simulink model "elevator"  (R2015b)
settings: Solver=FixedStepAuto  StartTime=0.0  StopTime=200  FixedStep=1  MaxStep=1  RelTol=1e-3
libraries: simulink x12
settings Model: Creator=DNikolaev  LastModifiedBy=DNikolaev

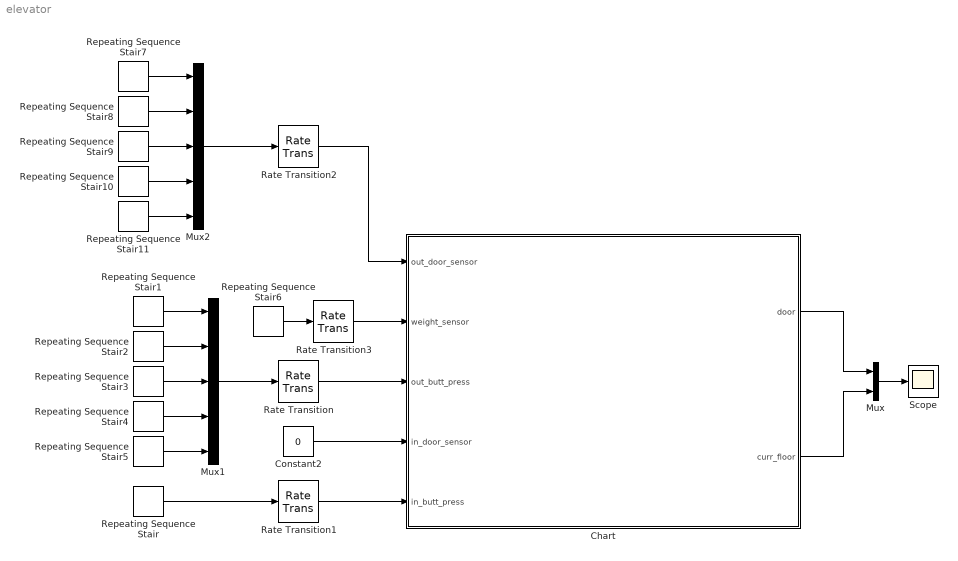
== system elevator ==
  Chart : Stateflow chart  TreatAsAtomicUnit=on
  Constant2 : Constant  Value=0
  Mux : Mux  Inputs=2
  Mux1 : Mux  Inputs=5
  Mux2 : Mux  Inputs=5
  Rate Transition{,1..3} (4 alike) : RateTransition  OutPortSampleTime=1
  Repeating Sequence Stair : simulink/Sources/Repeating Sequence Stair  OutValues=[0 0 0 4 0 0 0 0 0 1 0 0 0 0 0 0 0 0 0 0 0 0 0].'  tsamp=10  OutMin=[]  OutMax=[]  OutDataTypeStr=double  OutputDataTypeScalingMode=double  OutDataType=fixdt(0,8)  ConRadixGroup=Best Precision: Vector-wise  OutScaling=2^-12
  Repeating Sequence Stair1 : simulink/Sources/Repeating Sequence Stair  OutValues=[0 0 0 0 0 0 0 0 0 0 0 0 0 0 1 0 0 0 0 0].'  tsamp=10  OutMin=[]  OutMax=[]  OutDataTypeStr=double  OutputDataTypeScalingMode=double  OutDataType=fixdt(0,8)  ConRadixGroup=Best Precision: Vector-wise  OutScaling=2^-12
  Repeating Sequence Stair{3,5,7,9..11} (6 alike) : simulink/Sources/Repeating Sequence Stair  OutValues=[0 0 0 0 0 0 0 0 0 0 0 0 0 0 0 0 0 0 0 0].'  tsamp=10  OutMin=[]  OutMax=[]  OutDataTypeStr=double  OutputDataTypeScalingMode=double  OutDataType=fixdt(0,8)  ConRadixGroup=Best Precision: Vector-wise  OutScaling=2^-12
  Repeating Sequence Stair2 : simulink/Sources/Repeating Sequence Stair  OutValues=[0 1 0 0 0 0 0 0 0 0 0 0 0 0 0 0 0 0 0 0].'  tsamp=10  OutMin=[]  OutMax=[]  OutDataTypeStr=double  OutputDataTypeScalingMode=double  OutDataType=fixdt(0,8)  ConRadixGroup=Best Precision: Vector-wise  OutScaling=2^-12
  Repeating Sequence Stair4 : simulink/Sources/Repeating Sequence Stair  OutValues=[0 0 0 0 0 0 0 1 0 0 0 0 0 0 0 0 0 0 0 0].'  tsamp=10  OutMin=[]  OutMax=[]  OutDataTypeStr=double  OutputDataTypeScalingMode=double  OutDataType=fixdt(0,8)  ConRadixGroup=Best Precision: Vector-wise  OutScaling=2^-12
  Repeating Sequence Stair6 : simulink/Sources/Repeating Sequence Stair  OutValues=[0 0 0 50 0 0 0 0 400 400 400 200 200 0 0 0 0 0 0 0].'  tsamp=10  OutMin=[]  OutMax=[]  OutDataTypeStr=double  OutputDataTypeScalingMode=double  OutDataType=fixdt(0,8)  ConRadixGroup=Best Precision: Vector-wise  OutScaling=2^-12
  Repeating Sequence Stair8 : simulink/Sources/Repeating Sequence Stair  OutValues=[0 1 1 0 0 0 0 0 0 0 0 0 0 0 0 0 0 0 0 0].'  tsamp=10  OutMin=[]  OutMax=[]  OutDataTypeStr=double  OutputDataTypeScalingMode=double  OutDataType=fixdt(0,8)  ConRadixGroup=Best Precision: Vector-wise  OutScaling=2^-12
  Scope : Scope
  wires:
  Mux1/1 -> Rate Transition/1
  Constant2/1 -> Chart/4(in_door_sensor)
  Mux2/1 -> Rate Transition2/1
  Repeating Sequence Stair/1 -> Rate Transition1/1
  Chart/1(door) -> Mux/1
  Chart/2(curr_floor) -> Mux/2
  Mux/1 -> Scope/1
  Repeating Sequence Stair1/1 -> Mux1/1
  Repeating Sequence Stair2/1 -> Mux1/2
  Repeating Sequence Stair3/1 -> Mux1/3
  Repeating Sequence Stair4/1 -> Mux1/4
  Repeating Sequence Stair5/1 -> Mux1/5
  Rate Transition/1 -> Chart/3(out_butt_press)
  Rate Transition1/1 -> Chart/5(in_butt_press)
  Repeating Sequence Stair6/1 -> Rate Transition3/1
  Repeating Sequence Stair7/1 -> Mux2/1
  Repeating Sequence Stair10/1 -> Mux2/4
  Repeating Sequence Stair11/1 -> Mux2/5
  Rate Transition2/1 -> Chart/1(out_door_sensor)
  Rate Transition3/1 -> Chart/2(weight_sensor)
  Repeating Sequence Stair9/1 -> Mux2/3
  Repeating Sequence Stair8/1 -> Mux2/2

== stateflow chart elevator/Chart ==
  state Elevator [parallel]
    settings: executionOrder=1
    state Closed
      en: door=0
      state Wait
        en: state=1;
      state OpenRequest
      state Down
        en: state=3;
        move_down_mem=move_down;
        ex: curr_floor=curr_floor-move_down_mem;
      state Up
        en: state=2;
        move_up_mem=move_up;
        ex: curr_floor=curr_floor+move_up_mem;
      (default) -> Elevator.Closed.Wait
      Elevator.Closed.Wait -> OpenRequest [order 1] : [open_cmd==1]
      Up -> Elevator.Closed.Wait : [move_up==0]
      Elevator.Closed.Wait -> Up [order 2] : [move_up>0]
      Down -> Elevator.Closed.Wait : [move_down==0]
      Elevator.Closed.Wait -> Down [order 3] : [move_down>0]
    state Opened
      en:state=4;
      door=1;
      state Wait
      state CloseRequest
      Elevator.Opened.Wait -> CloseRequest : [close_cmd==1]
      CloseRequest -> Elevator.Opened.Wait [order 2] : [close_cmd==0]
    (default) -> Closed : {curr_floor=1;}
    OpenRequest -> Elevator.Opened.Wait : after(3,sec)
    CloseRequest -> Elevator.Closed.Wait [order 1] : after(3,sec)
  state InButtons [parallel]
    settings: executionOrder=2
    state Wait
      en: in_butt_state=0;
    state Pressed
      en: in_butt_state=in_butt_press;
      du: in_butt_state=in_butt_press;
    (default) -> InButtons.Wait : {in_butt_state=0;}
    InButtons.Wait -> Pressed : [in_butt_press>0]
    Pressed -> InButtons.Wait [order 2] : [in_butt_press==0]
    Pressed -> InButtons.Wait [order 1] : after(20,sec)
  state OutButtons [parallel]
    en: out_butt_state=0;
    but1=0;but2=0;but3=0;but4=0;but5=0;
    du: out_butt_state=out_button(but1,but2,but3,but4,but5)
    settings: executionOrder=3
    state Floor4 [parallel]
      settings: executionOrder=4
      state Wait1
      state Pressed1
        en: but4=1;
        ex: but4=0
      (default) -> OutButtons.Floor4.Wait1
      OutButtons.Floor4.Wait1 -> OutButtons.Floor4.Pressed1 : [out_butt_press(4)>0]
      OutButtons.Floor4.Pressed1 -> OutButtons.Floor4.Wait1 [order 1] : [state==4|| curr_floor==4]
      OutButtons.Floor4.Pressed1 -> OutButtons.Floor4.Wait1 [order 2] : after(100,sec)
    state Floor1 [parallel]
      settings: executionOrder=1
      state Wait1
      state Pressed1
        en: but1=1;
        ex: but1=0;
      (default) -> OutButtons.Floor1.Wait1
      OutButtons.Floor1.Wait1 -> OutButtons.Floor1.Pressed1 : [out_butt_press(1)>0]
      OutButtons.Floor1.Pressed1 -> OutButtons.Floor1.Wait1 [order 1] : [state==4|| curr_floor==1]
      OutButtons.Floor1.Pressed1 -> OutButtons.Floor1.Wait1 [order 2] : after(100,sec)
    state Floor2 [parallel]
      settings: executionOrder=2
      state Wait1
      state Pressed1
        en: but2=1;
        ex: but2=0
      (default) -> OutButtons.Floor2.Wait1
      OutButtons.Floor2.Wait1 -> OutButtons.Floor2.Pressed1 : [out_butt_press(2)>0]
      OutButtons.Floor2.Pressed1 -> OutButtons.Floor2.Wait1 [order 1] : [state==4|| curr_floor==2]
      OutButtons.Floor2.Pressed1 -> OutButtons.Floor2.Wait1 [order 2] : after(100,sec)
    state Floor3 [parallel]
      settings: executionOrder=3
      state Wait1
      state Pressed1
        en: but3=1;
        ex: but3=0
      (default) -> OutButtons.Floor3.Wait1
      OutButtons.Floor3.Wait1 -> OutButtons.Floor3.Pressed1 : [out_butt_press(3)>0]
      OutButtons.Floor3.Pressed1 -> OutButtons.Floor3.Wait1 [order 1] : [state==4|| curr_floor==3]
      OutButtons.Floor3.Pressed1 -> OutButtons.Floor3.Wait1 [order 2] : after(100,sec)
    state Floor5 [parallel]
      settings: executionOrder=5
      state Wait1
      state Pressed1
        en: but5=1;
        ex: but5=0
      (default) -> OutButtons.Floor5.Wait1
      OutButtons.Floor5.Wait1 -> OutButtons.Floor5.Pressed1 : [out_butt_press(5)>0]
      OutButtons.Floor5.Pressed1 -> OutButtons.Floor5.Wait1 [order 1] : [state==4|| curr_floor==5]
      OutButtons.Floor5.Pressed1 -> OutButtons.Floor5.Wait1 [order 2] : after(100,sec)
  state Comands [parallel]
    settings: executionOrder=4
    state Wait
    state Stay
    state MoveUp
      en:move_up=in_butt_state-curr_floor;
      ex:move_up=0;
    state MoveUp1
      en:move_up=out_butt_state-curr_floor;
      ex:move_up=0;
    state MoveDown
      en:move_down=curr_floor-in_butt_state;
      ex: move_down=0;
    state MoveDown1
      en:move_down=curr_floor-out_butt_state;
      ex: move_down=0;
    state OpenDoor
      en: open_cmd=1;
      ex: open_cmd=0;
    state CloseDoor
      en: close_cmd=1;
      ex: close_cmd=0;
    (default) -> Comands.Wait : {open_cmd=0;close_cmd=0;move_up=0;move_down=0}
    Comands.Wait -> (junction 64) [order 2] : [out_butt_state>0 && overweight(weight_sensor)==0]
    CloseDoor -> Comands.Wait [order 2] : [state==1]
    Stay -> Comands.Wait
    Comands.Wait -> (junction 53) [order 1] : [in_butt_state>0 && overweight(weight_sensor)==0 && underweight(weight_sensor)==0]
    (junction 53) -> Stay [order 2] : [in_butt_state==curr_floor]
    (junction 64) -> OpenDoor [order 3] : [out_butt_state==curr_floor]
    (junction 64) -> MoveDown1 [order 2] : [out_butt_state<curr_floor]
    (junction 64) -> MoveUp1 [order 1] : [out_butt_state>curr_floor]
    (junction 53) -> MoveUp [order 1] : [in_butt_state>curr_floor]
    (junction 53) -> MoveDown [order 3] : [in_butt_state<curr_floor]
    MoveUp -> OpenDoor : after(move_up*5,sec)
    MoveUp1 -> OpenDoor : after(move_up*5,sec)
    MoveDown -> OpenDoor : after(move_down*5,sec)
    MoveDown1 -> OpenDoor : after(move_down*5,sec)
    CloseDoor -> OpenDoor [order 1] : [in_door_sensor==1 || out_door_sensor(curr_floor)==1]
    OpenDoor -> CloseDoor : [state==4]
  data: b1 function_input; b2 function_input; b3 function_input; b4 function_input; b5 function_input; b function_output; ws function_input; under function_output; ws function_input; over function_output; out_door_sensor input; weight_sensor input; out_butt_press input; in_door_sensor input; in_butt_press input; door output; but1 local; but2 local; state local; move_up local; open_cmd local; but5 local; but3 local; but4 local; out_butt_state local; move_down local; close_cmd local; curr_floor output; in_butt_state local; move_up_mem local; move_down_mem local
  function b=out_button(b1,b2,b3,b4,b5):
    | function b=out_button(b1,b2,b3,b4,b5)
    |  if b1==1
    |      b=1;
    |  elseif b2==1
    |      b=2;
    |  elseif b3==1
    |      b=3;
    |  elseif b4==1
    |      b=4;
    |  elseif b5==1
    |      b=5;
    |  else
    |      b=0;
    |  end;
  function under=underweight(ws):
    | function under=underweight(ws)
    |     if ws<10
    |         under=1;
    |     else
    |         under=0;
    |     end
  function over=overweight(ws):
    | function over=overweight(ws)
    |     if ws>300
    |         over=1;
    |     else
    |         over=0;
    |     end
